simulink model "release_party"  (R2020a)
settings: Solver=VariableStepAuto  StartTime=0.0  StopTime=300  RelTol=1e-3
values from neighbouring files (symbols this model uses):
  n_beers = 19    [drinks.mat]    (also in release_party_mat.m = 20)
  n_drinks = 23    [drinks.mat]    (also in release_party_mat.m = 10)
  n_shots = 28    [drinks.mat]    (also in release_party_mat.m = 10)
  n_wines = 18    [drinks.mat]    (also in release_party_mat.m = 10)
  promille_beer = 1.31019577584    [drinks.mat]    (also in release_party_mat.m = SimOut.beer_promille.Data(length(out.beer_promille.Data)))
  promille_drink = 2.54699694719    [drinks.mat]    (also in release_party_mat.m = SimOut.drink_promille.Data(length(out.drink_promille.Data)))
  promille_shot = 8.39504310516    [drinks.mat]    (also in release_party_mat.m = SimOut.shot_promille.Data(length(out.shot_promille.Data)))
  promille_wine = 1.89552979079    [drinks.mat]    (also in release_party_mat.m = SimOut.wine_promille.Data(length(out.wine_promille.Data)))
settings Model: EnablePacing=on  Creator=tikjetsa  LastModifiedBy=tikjetsa

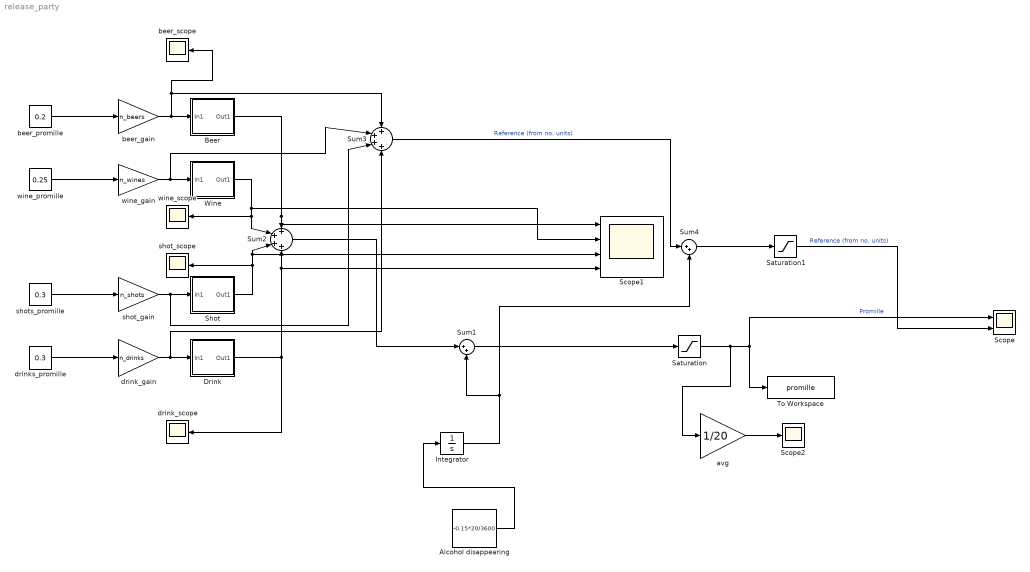
== system release_party ==
  Alcohol disappearing : Constant  Value=-0.15*20/3600
  Beer : Subsystem
  Drink : Subsystem
  Integrator : Integrator
  Saturation : Saturate  UpperLimit=inf  LowerLimit=0
  Saturation1 : Saturate  UpperLimit=inf  LowerLimit=0
  Scope : Scope  NumInputPorts=2
  Scope1 : Scope  NumInputPorts=4
  Scope2 : Scope
  Shot : Subsystem
  Sum1 : Sum  Inputs=|++
  Sum2 : Sum  Inputs=++++
  Sum3 : Sum  Inputs=++++
  Sum4 : Sum  Inputs=|++
  To Workspace : ToWorkspace  VariableName=promille  SaveFormat=Timeseries  SampleTime=1
  Wine : Subsystem
  avg : Gain  Gain=1/20
  beer_gain : Gain  Gain=n_beers
  beer_promille : Constant  Value=0.2
  beer_scope : Scope
  drink_gain : Gain  Gain=n_drinks
  drink_scope : Scope
  drinks_promille : Constant  Value=0.3
  shot_gain : Gain  Gain=n_shots
  shot_scope : Scope
  shots_promille : Constant  Value=0.3
  wine_gain : Gain  Gain=n_wines
  wine_promille : Constant  Value=0.25
  wine_scope : Scope
  wires:
  Alcohol disappearing/1 -> Integrator/1
  Integrator/1 -> Sum4/2, Sum1/2
  Sum1/1 -> Saturation/1
  wine_promille/1 -> wine_gain/1
  drinks_promille/1 -> drink_gain/1
  shots_promille/1 -> shot_gain/1
  beer_promille/1 -> beer_gain/1
  Sum2/1 -> Sum1/1
  Beer/1(Out1) -> Scope1/1, Sum2/1
  beer_gain/1 -> Sum3/1, beer_scope/1, Beer/1(In1)
  drink_gain/1 -> Sum3/4, Drink/1(In1)
  shot_gain/1 -> Sum3/3, Shot/1(In1)
  wine_gain/1 -> Sum3/2, Wine/1(In1)
  Wine/1(Out1) -> Sum2/2, wine_scope/1, Scope1/2
  Shot/1(Out1) -> Scope1/3, Sum2/3, shot_scope/1
  Drink/1(Out1) -> Sum2/4, Scope1/4, drink_scope/1
  Saturation/1 -> avg/1, Scope/1, To Workspace/1  "Promille"
  avg/1 -> Scope2/1
  Sum3/1 -> Sum4/1  "Reference (from no. units)"
  Sum4/1 -> Saturation1/1
  Saturation1/1 -> Scope/2  "Reference (from no. units)"

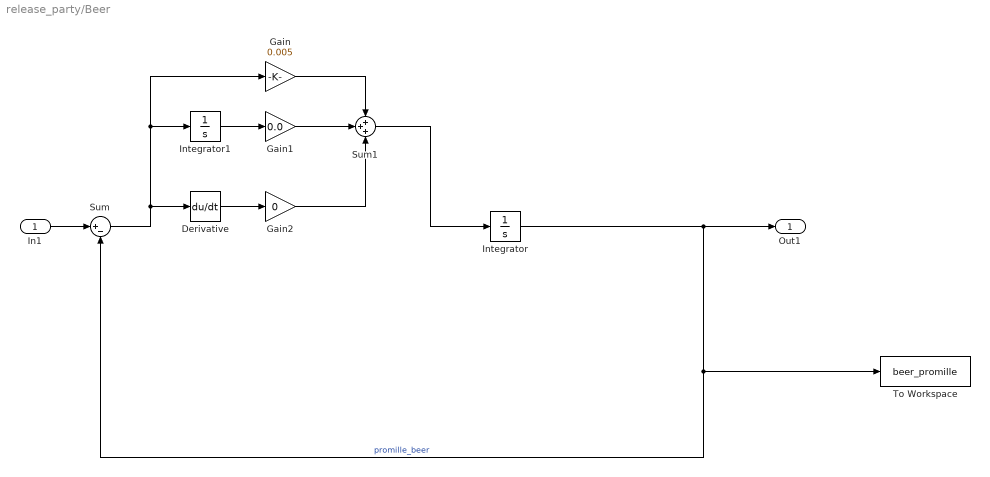
== system release_party/Beer ==
  In1 : Inport
  Derivative : Derivative
  Gain : Gain  Gain=0.005
  Gain1 : Gain  Gain=0.0
  Gain2 : Gain  Gain=0
  Integrator : Integrator  InitialCondition=promille_beer
  Integrator1 : Integrator
  Sum : Sum  Inputs=|+-
  Sum1 : Sum  Inputs=+++
  To Workspace : ToWorkspace  VariableName=beer_promille  SaveFormat=Timeseries  SampleTime=-1
      settings: MaxDataPoints=1
  Out1 : Outport
  wires:
  In1/1 -> Sum/1
  Sum1/1 -> Integrator/1
  Gain1/1 -> Sum1/2
  Gain/1 -> Sum1/1
  Integrator1/1 -> Gain1/1
  Sum/1 -> Derivative/1, Gain/1, Integrator1/1
  Gain2/1 -> Sum1/3
  Derivative/1 -> Gain2/1
  Integrator/1 -> To Workspace/1, Sum/2, Out1/1  "promille_beer"

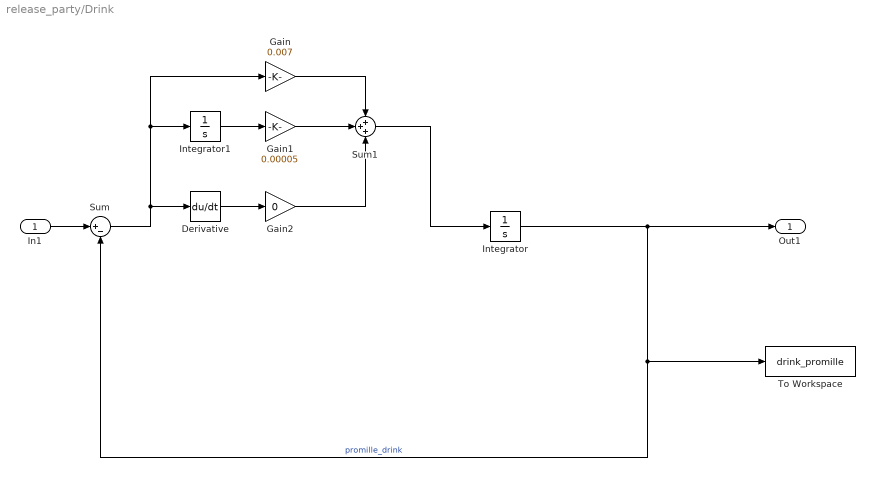
== system release_party/Drink ==
  In1 : Inport
  Derivative : Derivative
  Gain : Gain  Gain=0.007
  Gain1 : Gain  Gain=0.00005
  Gain2 : Gain  Gain=0
  Integrator : Integrator  InitialCondition=promille_drink
  Integrator1 : Integrator
  Sum : Sum  Inputs=|+-
  Sum1 : Sum  Inputs=+++
  To Workspace : ToWorkspace  VariableName=drink_promille  SaveFormat=Timeseries  SampleTime=-1
      settings: MaxDataPoints=1
  Out1 : Outport
  wires:
  In1/1 -> Sum/1
  Sum1/1 -> Integrator/1
  Gain1/1 -> Sum1/2
  Gain/1 -> Sum1/1
  Integrator/1 -> Out1/1, To Workspace/1, Sum/2  "promille_drink"
  Integrator1/1 -> Gain1/1
  Sum/1 -> Derivative/1, Gain/1, Integrator1/1
  Gain2/1 -> Sum1/3
  Derivative/1 -> Gain2/1

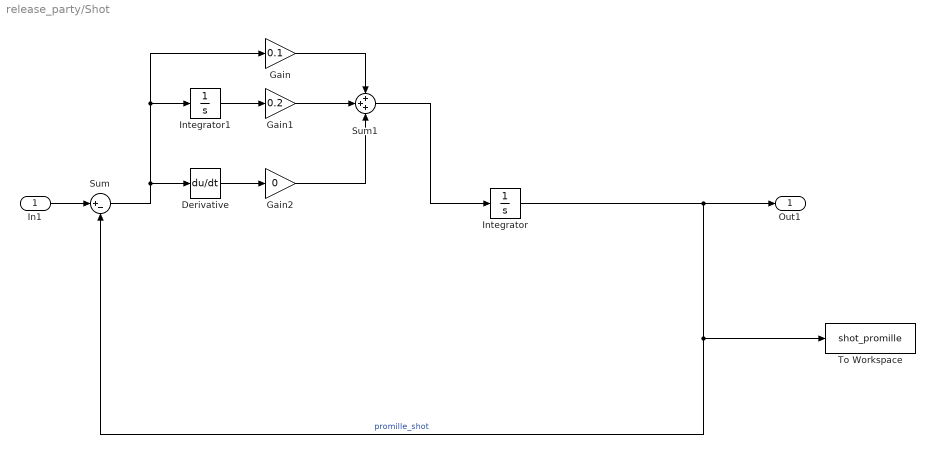
== system release_party/Shot ==
  In1 : Inport
  Derivative : Derivative
  Gain : Gain  Gain=0.1
  Gain1 : Gain  Gain=0.2
  Gain2 : Gain  Gain=0
  Integrator : Integrator  InitialCondition=promille_shot
  Integrator1 : Integrator
  Sum : Sum  Inputs=|+-
  Sum1 : Sum  Inputs=+++
  To Workspace : ToWorkspace  VariableName=shot_promille  SaveFormat=Timeseries  SampleTime=-1
      settings: MaxDataPoints=1
  Out1 : Outport
  wires:
  In1/1 -> Sum/1
  Sum1/1 -> Integrator/1
  Gain1/1 -> Sum1/2
  Gain/1 -> Sum1/1
  Integrator1/1 -> Gain1/1
  Sum/1 -> Derivative/1, Gain/1, Integrator1/1
  Gain2/1 -> Sum1/3
  Derivative/1 -> Gain2/1
  Integrator/1 -> To Workspace/1, Sum/2, Out1/1  "promille_shot"

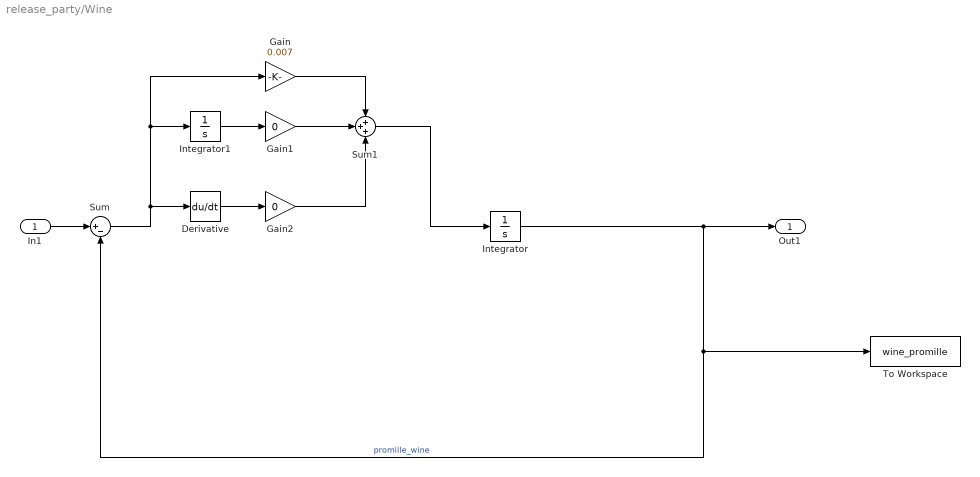
== system release_party/Wine ==
  In1 : Inport
  Derivative : Derivative
  Gain : Gain  Gain=0.007
  Gain1 : Gain  Gain=0
  Gain2 : Gain  Gain=0
  Integrator : Integrator  InitialCondition=promille_wine
  Integrator1 : Integrator
  Sum : Sum  Inputs=|+-
  Sum1 : Sum  Inputs=+++
  To Workspace : ToWorkspace  VariableName=wine_promille  SaveFormat=Timeseries  SampleTime=-1
      settings: MaxDataPoints=1
  Out1 : Outport
  wires:
  In1/1 -> Sum/1
  Sum1/1 -> Integrator/1
  Gain1/1 -> Sum1/2
  Gain/1 -> Sum1/1
  Integrator1/1 -> Gain1/1
  Sum/1 -> Derivative/1, Gain/1, Integrator1/1
  Gain2/1 -> Sum1/3
  Derivative/1 -> Gain2/1
  Integrator/1 -> To Workspace/1, Sum/2, Out1/1  "promille_wine"
